simulink model "ball_bahn2"  (Simulink 4.00)
settings: Solver=ode45  StartTime=0.0  StopTime=10.0  MaxStep=0.1  RelTol=1e-3
settings Model: LastModifiedBy=Administrator  Refine=3  BlockReductionOpt=off

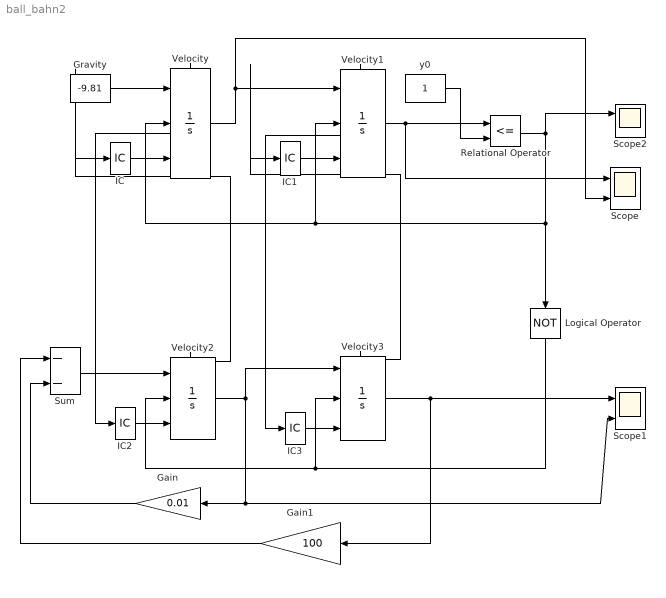
== system ball_bahn2 ==
  Gain : Gain  Orientation=left  Gain=0.01  Multiplication=Element-wise(K.*u)  SaturateOnIntegerOverflow=on
  Gain1 : Gain  Orientation=left  Gain=100  Multiplication=Element-wise(K.*u)  SaturateOnIntegerOverflow=on
  Gravity : Constant  Value=-9.81
  IC : InitialCondition  Value=0
  IC1 : InitialCondition  Value=15
  IC2 : InitialCondition  Value=0
  IC3 : InitialCondition  Value=0
  Logical Operator : Logic  Orientation=down  Operator=NOT  Inputs=2
  Relational Operator : RelationalOperator  Operator=<=
  Scope : Scope  NumInputPorts=2
      settings: TickLabels=on  TimeRange=auto  YMin=-30~0  YMax=20~22.9822  SaveToWorkspace=off  SaveName=ScopeData  DataFormat=Array  LimitDataPoints=on  MaxDataPoints=5000
  Scope1 : Scope  NumInputPorts=2
      settings: TickLabels=on  TimeRange=auto  YMin=-30~0  YMax=20~22.9822  SaveToWorkspace=off  DataFormat=Array  LimitDataPoints=on  MaxDataPoints=5000
  Scope2 : Scope  NumInputPorts=2
      settings: TimeRange=auto  YMin=-5~-5  YMax=5~5  SaveToWorkspace=off  SaveName=ScopeData2  LimitDataPoints=on  MaxDataPoints=5000
  Sum : Sum  Inputs=--  SaturateOnIntegerOverflow=on
  Velocity{,1..3} (4 alike) : Integrator  ExternalReset=level  InitialConditionSource=external  InitialCondition=0  LimitOutput=off  UpperSaturationLimit=inf  LowerSaturationLimit=-inf  ShowSaturationPort=off  ShowStatePort=on  AbsoluteTolerance=auto
  y0 : Constant  Value=1
  wires:
  Gravity/1 -> Velocity/1
  Velocity/1 -> Velocity1/1, Scope/2
  IC/1 -> Velocity/3
  IC1/1 -> Velocity1/3
  Velocity2/1 -> Gain/1, Scope1/2, Velocity3/1
  Velocity1/1 -> Relational Operator/1, Scope/1
  Velocity3/1 -> Gain1/1, Scope1/1
  Sum/1 -> Velocity2/1
  Gain/1 -> Sum/2
  Gain1/1 -> Sum/1
  y0/1 -> Relational Operator/2
  Relational Operator/1 -> Scope2/1, Velocity/2, Velocity1/2, Logical Operator/1
  IC2/1 -> Velocity2/3
  IC3/1 -> Velocity3/3
  Velocity2/State -> IC/1
  Velocity3/State -> IC1/1
  Velocity1/State -> IC3/1
  Velocity/State -> IC2/1
  Logical Operator/1 -> Velocity2/2, Velocity3/2
